simulink model "Rotor"  (R2023a)
settings: Solver=VariableStepAuto  StartTime=0.0  StopTime=1  RelTol=1e-3
libraries: simulink x1, aerolibpropulsion2 x1
settings Model: Creator=vboutrou  LastModifiedBy=vboutrou

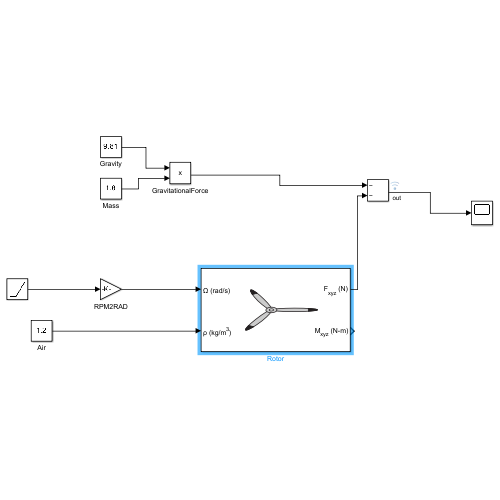
[thumbnail: Simulink's stored preview of the top-level diagram]
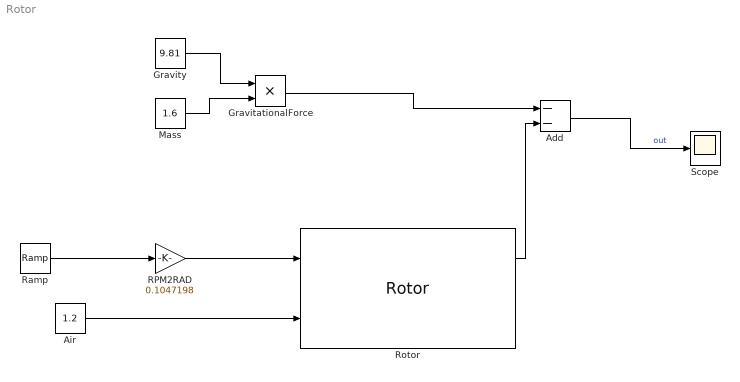
== system Rotor ==
  Add : Sum  Inputs=--
  Air : Constant  Value=1.2
  GravitationalForce : Product  Inputs=**
  Gravity : Constant  Value=9.81
  Mass : Constant  Value=1.6
  RPM2RAD : Gain  Gain=0.1047198
  Ramp : simulink/Sources/Ramp  slope=3500  start=0  InitialOutput=0
  Rotor : aerolibpropulsion2/Rotor  units=Metric (MKS)  modelMode=Without flap effects  blockSelect=Single  config=Quadcopter X  Nr=1  l=0.0624  h=-0.0159  Arm=[0;0;0]  Nb=2  CTcheck=off  CT=0.0107  CQ=7.8263e-4  CTout=off  R=1  c=0.0080  e=0  clalpha=5.5  gamma=0.6051  twistType=Linear  theta0=0.2548  theta1=-0.1361  thetaTip=0.1018  Vb=[0;0;0]  pqr=[0;0;0]
      settings: LibrarySourceBlock=aerolibrotor/Rotor
  Scope : Scope
  wires:
  RPM2RAD/1 -> Rotor/1
  Air/1 -> Rotor/2
  Gravity/1 -> GravitationalForce/1
  Mass/1 -> GravitationalForce/2
  GravitationalForce/1 -> Add/1
  Rotor/1 -> Add/2
  Ramp/1 -> RPM2RAD/1
  Add/1 -> Scope/1  "out"
